simulink model "Estimator_Simulink"  (R2019a)
settings: Solver=VariableStepAuto  StartTime=0.0  StopTime=90000  RelTol=1e-3
InitFcn:
  | load('Sim_Truth_SecondOrder_Corrected5.mat')
values from neighbouring files (symbols this model uses):
  A = [-1/(Rc*Cc) 0; 0 0]    [BatteryModel_1stOrder_Youla.m]    (also in Estimator_Simulink_driver.m = [1 0 ; 0 (1-(dt/(Rc*Cc)))]; battery_equivalent_circuit_model_KF.m = 1)
  B = [1/Cc; -1/Cbat]    [BatteryModel_1stOrder_Youla.m]    (also in Estimator_Simulink_driver.m = [-(dt/Cbat) ; (dt/Cc)]; battery_equivalent_circuit_model_KF.m = -5.55555555556e-06)
  C = [-1 alpha]    [BatteryModel_1stOrder_Youla.m]    (also in Estimator_Simulink_driver.m = [alpha -1]; battery_equivalent_circuit_model_KF.m = 0.65)
  D = -R0    (= -0.1)    [BatteryModel_1stOrder_Youla.m]    (also in Estimator_Simulink_driver.m = [-R0]; battery_equivalent_circuit_model_KF.m = -0.01)
undefined symbols (not defined in the file or in its folder): den, num
libraries: dspsrcs4 x1, dspstat3 x1
settings Model: Creator=Indiana  LastModifiedBy=felip
settings DataIOCC: ReturnWorkspaceOutputs=off
settings DebuggingCC: ArithmeticOperatorsInVariantConditions=warning

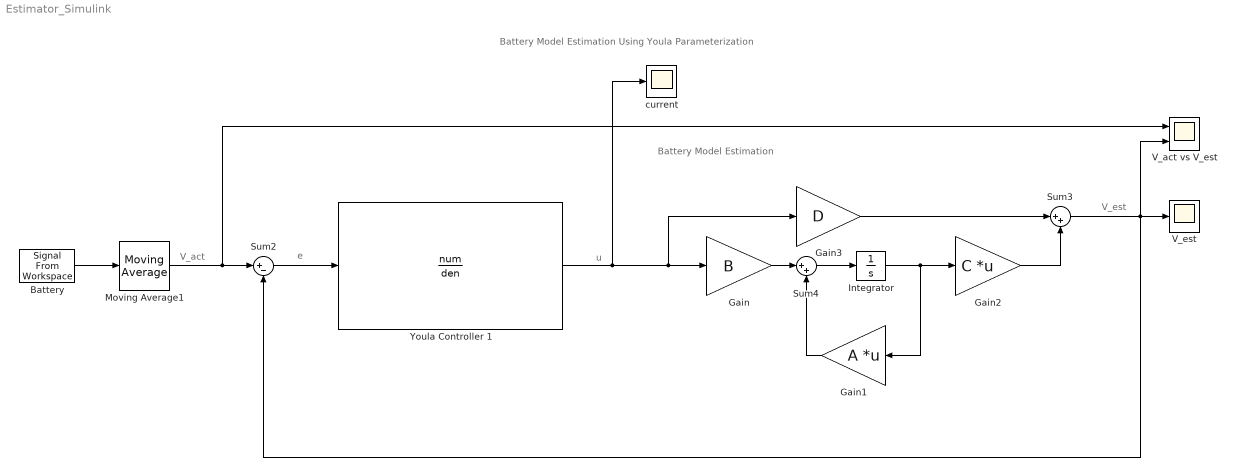
== system Estimator_Simulink ==
  note: Battery Model Estimation Using Youla Parameterization
  note: V_act
  note: V_est
  note: u
  note: e
  note: Battery Model Estimation
  Battery : dspsrcs4/Signal From Workspace  X=V  Ts=1  nsamps=1  OutputAfterFinalValue=Setting to zero  ignoreOrWarnInputAndFrameLengths=off  OutputFrames=off
  Gain : Gain  Gain=B
  Gain1 : Gain  Gain=A  Multiplication=Matrix(K*u)
  Gain2 : Gain  Gain=C  Multiplication=Matrix(K*u)
  Gain3 : Gain  Gain=D
  Integrator : Integrator  InitialCondition=[3.345;.98]
  Moving Average1 : dspstat3/Moving Average  Method=Sliding window  ForgettingFactorPort=off  SpecifyWindowLength=on  WindowLength=15  ForgettingFactor=0.9  SimulateUsing=Code generation
  Sum2 : Sum  Inputs=|+-
  Sum3 : Sum  Inputs=|++
  Sum4 : Sum  Inputs=|++
  V_act vs V_est : Scope  NumInputPorts=2
  "V_est " : Scope
  Youla Controller 1 : TransferFcn  Numerator=num  Denominator=den
  "current " : Scope
  wires:
  Moving Average1/1 -> V_act vs V_est/1, Sum2/1
  Battery/1 -> Moving Average1/1
  Sum2/1 -> Youla Controller 1/1
  Sum3/1 -> "V_est "/1, Sum2/2, V_act vs V_est/2
  Youla Controller 1/1 -> "current "/1, Gain3/1, Gain/1
  Gain3/1 -> Sum3/1
  Gain2/1 -> Sum3/2
  Gain1/1 -> Sum4/2
  Sum4/1 -> Integrator/1
  Integrator/1 -> Gain1/1, Gain2/1
  Gain/1 -> Sum4/1
